simulink model "L4_SIM"  (R2018a)
settings: Solver=ode1  StartTime=0.0  StopTime=60  FixedStep=GLB_FIXED_STEP_SIZE_CPV  RelTol=1e-3  EnableMultiTasking=on
undefined symbols (not defined in the file or in its folder): Cf, Chassis, Cr, CYCLE_ACC1_2A__AdaptiveCruiseCtrlMode, CYCLE_ACC1_2A__AdaptiveCruiseCtrlSetSpeed, CYCLE_CCVS1_00__CruiseCtrlSetSpeed, CYCLE_CCVS1_00__WheelBasedVehicleSpeed, CYCLE_EEC1_00__EngSpeed, CYCLE_ETC1_00__TransDrivelineEngaged, CYCLE_ETC2_00__TransActualGearRatio, CYCLE_ETC7_03__TransMode1Indicator, CYCLE_GPS_Latitude, CYCLE_GPS_Longitude, CYCLE_LFE1_00__EngFuelRate, CYCLE_Net_Engine_Percent_Torque, CYCLE_SSI2_03__PitchAngleExRange, CYCLE_TIME, CYCLE_UTM_Origin_X, CYCLE_UTM_Origin_Y, CYCLE_Vehicle_Distance, DiscIntNeverNeededParam, ENUM_J1939_PCC_STATE_T, ENUM_J1939_SWITCH_T, ENUM_STEERING_WHEEL_ANGLE_SENSOR_TYPE_T, GLB_FIXED_STEP_SIZE_CPV, GLB_TRANS_LOSS_TRQ_GEAR_STEP_MPV, GLB_TRANS_LOSS_TRQ_SPD_STEP_MPV, GLB_TRANS_LOSS_TRQ_TABLE_DATA_MPV, GLB_TRANS_LOSS_TRQ_TRQ_STEP_MPV, GLB_VEHICLE_CONFIG_ACCEL_PED_GATEWAY_APV, heading_0, Iz, L4_Controller, lf, lr, position_0, ptc_matlab_lib, STEERCTRL_10ms, SUB_ECU_L4_MABX, SUB_L4_Task_10ms, SUB_L4_Task_10ms_SUB_STEERCTRL, SUB_PLANT_Chassis, Task_10ms, Vx_0
libraries: EmE_MBD_Blockset x81, PTC_MBDS_LIB x71, simulink x38, simulink_extras x1, SUB_L4_Task_10000ms x1, SUB_L4_Task_1000ms x1, SUB_L4_Task_100ms x1, SUB_L4_Task_10ms_SUB_APTC x1, SUB_L4_Task_10ms_SUB_BRKPEDARB x1, SUB_L4_Task_10ms_SUB_FAULT_MANAGER x1, SUB_L4_Task_10ms_SUB_STATE_CONTROL x1, simulink_need_slupdate x1
(part 2 of 6)

== system L4_SIM/Controllers/Virtual_Controllers/VECU ==
  In1 : Inport
  Bus Creator1 : BusCreator  Inputs=1
  Bus Creator2 : BusCreator  Inputs=2
  Constant1 : Constant  Value=0
  Constant2 : Constant  Value=0
  Terminator : Terminator
  Out1 : Outport
  wires:
  Bus Creator1/1 -> Out1/1
  In1/1 -> Terminator/1
  Bus Creator2/1 -> Bus Creator1/1  "TSC1_P4_VECU"
  Constant2/1 -> Bus Creator2/2  "TrqReq"
  Constant1/1 -> Bus Creator2/1  "OCM"

== system L4_SIM/Controllers/Virtual_Controllers/VEMC ==
  In1 : Inport
  Bus Creator1 : BusCreator  Inputs=3
  Bus Creator2 : BusCreator  Inputs=2
  Bus Creator3 : BusCreator  Inputs=2
  Constant{1..4} (4 alike) : Constant  Value=0
  Constant5 : Constant  Value=false
  Terminator : Terminator
  Out1 : Outport
  wires:
  Bus Creator1/1 -> Out1/1
  In1/1 -> Terminator/1
  Bus Creator2/1 -> Bus Creator1/1  "TSC1_P2_VEMCE"
  Constant2/1 -> Bus Creator2/2  "TrqReqE"
  Constant1/1 -> Bus Creator2/1  "OCME"
  Constant3/1 -> Bus Creator3/1  "OCMR"
  Constant4/1 -> Bus Creator3/2  "TrqReqR"
  Bus Creator3/1 -> Bus Creator1/2  "TSC1_P32_VEMCR"
  Constant5/1 -> Bus Creator1/3  "NeutralCoastRequest"

== system L4_SIM/Plant/PlantModel/Chassis ==
  Engine : Inport
  FoundationBrakes : Inport  Port=2
  AMT : Inport  Port=3
  Cycle : Inport  Port=4
  ABS : Inport  Port=5
  L4_MABX : Inport  Port=6
  Navigation : Inport  Port=7
  Bus Creator : BusCreator  Inputs=51
  Bus Selector : BusSelector  OutputSignals=EngineFricTrq,EngineIndicatedTrq,RetarderActTrqDem,RetarderTrqMax,EngFuelRate_lph,EngineIndicatedTrqMax,EngActNetTrqPer,EngActFricTrqPer,EngActIndTrqPer
  Bus Selector1 : BusSelector  OutputSignals=PitchAngle
  Bus Selector2 : BusSelector  OutputSignals=ShiftControl.Internal.GearNumberCommand,ShiftControl.Internal.MainClutch
  Bus Selector3 : BusSelector  OutputSignals=AeroDragForce,InclineForce,TireDragForce,TireResistancePower,RetarderNetTrq,RetarderPercentTrq,VehAccel,Vy,Yaw Rate
  Bus Selector4 : BusSelector  OutputSignals=ABS_VEHICLE_MASS_APV
  Bus Selector5 : BusSelector  OutputSignals=10msTask.SteeringControl.DesSteeringAngle
  Bus Selector6 : BusSelector  OutputSignals=Navigation.VehHeading
  Chassis_SL : Subsystem
  Constant : PTC_MBDS_LIB/Extras/Sources/Constant  Value2=GLB_AIR_DENSITY_APV  PTC_MBDS_BlockVersion=5.41  PTC_BlockType=PTC_MBDS_Constant
      settings: SourceProductName=PACCAR Technical Center MBDS Library
      settings: AttributesFormatString=|
      | Value: 1.23696005344
      | Unit: 'kg/m^3'
  Constant1 : PTC_MBDS_LIB/Extras/Sources/Constant  Value2=GLB_AXLE_EFFICIENCY_APV  PTC_MBDS_BlockVersion=5.41  PTC_BlockType=PTC_MBDS_Constant
      settings: SourceProductName=PACCAR Technical Center MBDS Library
      settings: AttributesFormatString=|
      | Value: 0.980000019073
      | Unit: '1'
  Constant11 : Constant  Value=[1,0]
  Constant2 : Constant  Value=[0 0]
  Constant3 : PTC_MBDS_LIB/Extras/Sources/Constant  Value2=GLB_CHASSIS_DRAG_COEFFICIENT_APV  PTC_MBDS_BlockVersion=5.41  PTC_BlockType=PTC_MBDS_Constant
      settings: SourceProductName=PACCAR Technical Center MBDS Library
      settings: AttributesFormatString=|
      | Value: 0.65
      | Unit: '1'
  Constant4 : Constant  Value=0
  Constant5 : Constant
  Constant9 : Constant  Value=[1,0]
  SignalConversion1 : SignalConversion  ConversionOutput=Contiguous copy  OverrideOpt=off
  SignalConversion3 : SignalConversion  ConversionOutput=Contiguous copy  OverrideOpt=off
  ChassisMdl_O : Outport
  wires:
  Bus Selector5/1 -> Chassis_SL/15(SteerAngle)  "<DesSteeringAngle>"
  L4_MABX/1 -> Bus Selector5/1
  Bus Selector3/9 -> Bus Creator/30  "<Yaw Rate>"
  Bus Selector3/8 -> Bus Creator/29  "<Vy>"
  Chassis_SL/28(BrakeSecondaryPressure_kpa) -> Bus Creator/36  "BrakeSecondaryPressure_kpa"
  Chassis_SL/27(BrakePrimaryPressure_kpa) -> Bus Creator/35  "BrakePrimaryPressure_kpa"
  Chassis_SL/26(BrakeApplicationPressure_kpa) -> Bus Creator/34  "BrakeApplicationPressure_kpa"
  Constant4/1 -> Chassis_SL/8(MotorTorqueRequest)
  SignalConversion1/1 -> Bus Creator/44  "EngineTorque_in"
  SignalConversion3/1 -> Bus Creator/43  "EngineFriction_In"
  Bus Selector/9 -> Bus Creator/51  "<EngActIndTrqPer>"
  Chassis_SL/21(VEHICLE_SPEED_OUT) -> Bus Creator/21  "VehicleSpeed"
  Chassis_SL/15(TRANSMISSION_SPEED_OUT) -> Bus Creator/15  "TransmissionSpeed"
  Bus Selector4/1 -> Chassis_SL/14(VehicleMass)  "<ABS_VEHICLE_MASS_APV>"
  ABS/1 -> Bus Selector4/1
  Constant/1 -> Chassis_SL/1(AirDensity)  "GLB_AIR_DENSITY_APV"
  Bus Selector/6 -> Bus Creator/48  "<EngineIndicatedTrqMax>"
  Bus Selector3/3 -> Bus Creator/24  "<TireDragForce>"
  Bus Selector/5 -> Bus Creator/47  "<EngFuelRate_lph>"
  Bus Selector3/7 -> Bus Creator/28  "<VehAccel>"
  Bus Selector/4 -> Bus Creator/46  "<RetarderTrqMax>"
  Bus Selector/3 -> Bus Creator/45  "<RetarderActTrqDem>"
  Bus Selector3/6 -> Bus Creator/27  "<RetarderPercentTrq>"
  Bus Selector/2 -> SignalConversion1/1  "<EngineIndicatedTrq>"
  Bus Selector/1 -> SignalConversion3/1  "<EngineFricTrq>"
  [Engine] -> Bus Selector/1
  Engine/1 -> Chassis_SL/7(EngineData), [Engine]
  Bus Selector3/5 -> Bus Creator/26  "<RetarderNetTrq>"
  Bus Selector3/4 -> Bus Creator/25  "<TireResistancePower>"
  Bus Selector3/2 -> Bus Creator/23  "<InclineForce>"
  Bus Selector3/1 -> Bus Creator/22  "<AeroDragForce>"
  Chassis_SL/22(DataBus) -> Bus Selector3/1  "ChassisDynamics"
  Chassis_SL/2(AXLE_SPEEDS_OUT[4]) -> Bus Creator/2  "AxleSpeeds"
  Bus Selector/8 -> Bus Creator/50  "<EngActFricTrqPer>"
  Bus Selector/7 -> Bus Creator/49  "<EngActNetTrqPer>"
  [FoundationBrakes] -> Bus Creator/37  "FoundationBrakes"
  FoundationBrakes/1 -> Chassis_SL/4(Brakes_Act), [FoundationBrakes]  "BrkDrv"
  AMT/1 -> Bus Selector2/1
  Bus Selector1/1 -> Chassis_SL/11(RoadAngle), Bus Creator/40  "<PitchAngle>"
  Cycle/1 -> Bus Selector1/1
  Chassis_SL/17(TRANSMISSION_TORQUE_OUT) -> Bus Creator/17  "TransmissionTorque"
  Chassis_SL/16(TRANSMISSION_STATE_LOCK_OUT) -> Bus Creator/16  "TransmissionStateLock"
  Chassis_SL/13(MEASURED_VEHICLE_SPEED_OUT) -> Bus Creator/13  "MeasuredVehicleSpeed_kph"
  Chassis_SL/12(MAIN_CLUTCH_LOCK_OUT) -> Bus Creator/12  "MainClutchLock"
  Chassis_SL/10(GEAR_NUMBER_OUT) -> Bus Creator/10  "GearNumber"
  Chassis_SL/9(ENGINE_RPM_OUT) -> Bus Creator/9  "EngineRPM"
  Chassis_SL/1(AXLE_POWER_LOSSES_OUT[2]) -> Bus Creator/1  "AxlePowerLosses"
  Bus Creator/1 -> ChassisMdl_O/1
  Bus Selector2/2 -> Chassis_SL/10(MainClutchAct), Bus Creator/39  "<MainClutch>"
  Constant2/1 -> Bus Creator/41, Chassis_SL/12(TransmissionLoss[2])  "TransmisisonLoss_In"
  Constant11/1 -> Bus Creator/42, Chassis_SL/13(TransmissionSpinLoss[2])  "TransSpinLoss_In"
  Constant9/1 -> Chassis_SL/6(DriveShaftLoss[2])
  Constant3/1 -> Chassis_SL/5(C_Drag)  "GLB_CHASSIS_DRAG_COEFFICIENT_APV"
  Constant5/1 -> Chassis_SL/3(Axle_Act_Lock)
  Constant1/1 -> Chassis_SL/2(AxleEff)  "GLB_AXLE_EFFICIENCY_APV"
  Chassis_SL/14(TRANSMISSION_POWER_LOSS_OUT) -> Bus Creator/14  "TransmissionPowerLoss"
  Chassis_SL/8(DRIVE_SHAFT_TORQUE_OUT) -> Bus Creator/8  "DriveShaftTorque"
  Chassis_SL/20(BrakeTrqRequest) -> Bus Creator/20  "ChassisBrakeTrqRequest"
  Chassis_SL/6(DRIVE_SHAFT_POWER_LOSS_OUT) -> Bus Creator/6  "DrIveShaftPowerLoss"
  Chassis_SL/18(TRANS_SPIN_POWER_LOSS_OUT) -> Bus Creator/18  "TransmissionSpinPowerLoss"
  Chassis_SL/4(BRAKES_LOCK_OUT[4]) -> Bus Creator/4  "BrakesLock"
  Chassis_SL/7(DRIVE_SHAFT_SPEED_OUT) -> Bus Creator/7  "DriveShaftSpeed"
  Chassis_SL/19(TRANS_SPIN_SPEED_OUT) -> Bus Creator/19  "TransmissionSpinSpeed"
  Chassis_SL/3(AXLE_TORQUES_OUT[2]) -> Bus Creator/3  "AxleTorques"
  Chassis_SL/11(GEAR_RATIO_OUT) -> Bus Creator/11  "GearRatio"
  Chassis_SL/5(DRIVE_AXLE_LOCK_OUT) -> Bus Creator/5  "DriveAxleLock"
  Bus Selector2/1 -> Bus Creator/38, Chassis_SL/9(GearNumber)  "<GearNumberCommand>"
  Chassis_SL/23(TrqFromClutch) -> Bus Creator/31  "TrqFromClutch"
  Chassis_SL/24(ClutchState) -> Bus Creator/32  "ClutchState"
  Chassis_SL/25(EngSpdClutchClosed) -> Bus Creator/33  "EngSpdClutchClosed"
  Navigation/1 -> Bus Selector6/1
  Bus Selector6/1 -> Chassis_SL/16(Heading)  "<VehHeading>"

== system L4_SIM/Plant/PlantModel/Navigation ==
  In1 : Inport
  Body velocity : Scope  NumInputPorts=2
  Bus Creator : BusCreator  Inputs=3
  Bus Selector : BusSelector  OutputSignals=VehicleSpeed,Vy,Yaw Rate
  Gain : Gain  Gain=180/pi
  Gain1 : Gain  Gain=1/3.6
  Heading : Scope  NumInputPorts=2
  Initial Heading : Constant  Value=heading_0
  Initial Position : Constant  Value=position_0
  Integrator : Integrator  InitialConditionSource=external
  Integrator2 : Integrator  InitialCondition=heading_0  UpperSaturationLimit=pi  LowerSaturationLimit=-pi  WrapState=on  WrappedStateUpperValue=2*pi  WrappedStateLowerValue=0
  MATLAB Function1 : MATLAB Function  TreatAsAtomicUnit=on
  Position : Scope
  Yaw rate : Scope
  Out1 : Outport
  wires:
  Gain1/1 -> MATLAB Function1/1(Vx), Body velocity/1
  Integrator2/1 -> MATLAB Function1/3(heading), Gain/1, Heading/1
  Gain/1 -> Bus Creator/3  "VehHeading"
  Integrator/1 -> Bus Creator/2, Position/1  "VehPosition"
  Bus Creator/1 -> Out1/1
  Initial Heading/1 -> Heading/2
  Initial Position/1 -> Integrator/2
  MATLAB Function1/1(Vnav) -> Integrator/1, Bus Creator/1  "VehVelNav"
  Bus Selector/2 -> MATLAB Function1/2(Vy), Body velocity/2  "<Vy>"
  Bus Selector/1 -> Gain1/1  "<VehicleSpeed>"
  Bus Selector/3 -> Integrator2/1, Yaw rate/1  "<Yaw Rate>"
  In1/1 -> Bus Selector/1

== system L4_SIM/Controllers/Drive_Cycle/DriveCycle/CruiseSetSpeedOverride ==
  SimActiveTime : Inport
  CCSetSpeed : Inport  Port=2
  Constant1 : PTC_MBDS_LIB/Extras/Sources/Constant  Value2=60  PTC_MBDS_BlockVersion=5.41  PTC_BlockType=PTC_MBDS_Constant
      settings: SourceProductName=PACCAR Technical Center MBDS Library
  Constant2 : PTC_MBDS_LIB/Extras/Sources/Constant  Value2=0  PTC_MBDS_BlockVersion=5.41  PTC_BlockType=PTC_MBDS_Constant
      settings: SourceProductName=PACCAR Technical Center MBDS Library
  Display : Display
  Display1 : Display
  If_Then_Else1 : PTC_MBDS_LIB/Extras/Signal Routing/If_Then_Else  PTC_MBDS_BlockVersion=5.41  PTC_BlockType=PTC_MBDS_If_Then_Else
      settings: SourceProductName=PACCAR Technical Center MBDS Library
  LE : PTC_MBDS_LIB/MBDS Standard Library/Basic Operations/Logic and Bit Operations/LE  InputSameDT=on  PTC_MBDS_BlockVersion=5.41  PTC_BlockType=PTC_MBDS_LE
      settings: SourceProductName=PACCAR Technical Center MBDS Library
  Out1 : Outport
  wires:
  Constant1/1 -> LE/2
  CCSetSpeed/1 -> If_Then_Else1/3
  SimActiveTime/1 -> Display/1, LE/1
  Constant2/1 -> If_Then_Else1/2
  If_Then_Else1/1 -> Display1/1, Out1/1
  LE/1 -> If_Then_Else1/1

== system L4_SIM/Controllers/Drive_Cycle/DriveCycle/CycleCalculations ==
  Actual_Vehicle_Speed[m/s] : Inport
  Discrete-Time Integrator : DiscreteIntegrator  IntegratorMethod=Integration: Trapezoidal  SampleTime=-1  ICPrevOutput=DiscIntNeverNeededParam  ICPrevScaledInput=DiscIntNeverNeededParam
  Saturation : Saturate  UpperLimit=Inf  LowerLimit=0
  Vehicle_Distance[m] : Outport
  wires:
  Actual_Vehicle_Speed[m/s]/1 -> Saturation/1
  Discrete-Time Integrator/1 -> Vehicle_Distance[m]/1
  Saturation/1 -> Discrete-Time Integrator/1

== system L4_SIM/Controllers/Operator/Subsystem/Gains ==
  note: These Gains should be the same for Acc Pedal
      | and Brake Pedal on the dyno
  Constant : PTC_MBDS_LIB/Extras/Sources/Constant  Value2=OPERATOR_Kp_Acc  PTC_MBDS_BlockVersion=5.41  PTC_BlockType=PTC_MBDS_Constant
      settings: SourceProductName=PACCAR Technical Center MBDS Library
      settings: AttributesFormatString=|
      | Value: 0.25
      | Unit: '1'
  Constant1 : PTC_MBDS_LIB/Extras/Sources/Constant  Value2=OPERATOR_Ti_Acc  PTC_MBDS_BlockVersion=5.41  PTC_BlockType=PTC_MBDS_Constant
      settings: SourceProductName=PACCAR Technical Center MBDS Library
      settings: AttributesFormatString=|
      | Value: 0.45
      | Unit: 's'
  Constant2 : PTC_MBDS_LIB/Extras/Sources/Constant  Value2=OPERATOR_Td_Acc  PTC_MBDS_BlockVersion=5.41  PTC_BlockType=PTC_MBDS_Constant
      settings: SourceProductName=PACCAR Technical Center MBDS Library
      settings: AttributesFormatString=|
      | Value: 0
      | Unit: 's'
  Constant3 : PTC_MBDS_LIB/Extras/Sources/Constant  Value2=OPERATOR_Kp_Brk  PTC_MBDS_BlockVersion=5.41  PTC_BlockType=PTC_MBDS_Constant
      settings: SourceProductName=PACCAR Technical Center MBDS Library
      settings: AttributesFormatString=|
      | Value: 0.38
      | Unit: '1'
  Constant4 : PTC_MBDS_LIB/Extras/Sources/Constant  Value2=OPERATOR_Ti_Brk  PTC_MBDS_BlockVersion=5.41  PTC_BlockType=PTC_MBDS_Constant
      settings: SourceProductName=PACCAR Technical Center MBDS Library
      settings: AttributesFormatString=|
      | Value: 0.25
      | Unit: 's'
  Constant5 : PTC_MBDS_LIB/Extras/Sources/Constant  Value2=OPERATOR_Td_Brk  PTC_MBDS_BlockVersion=5.41  PTC_BlockType=PTC_MBDS_Constant
      settings: SourceProductName=PACCAR Technical Center MBDS Library
      settings: AttributesFormatString=|
      | Value: 0
      | Unit: 's'
  Mux : Mux  Inputs=3
  Mux1 : Mux  Inputs=3
  Gains_Acc : Outport
  Gains_Brk : Outport  Port=2
  wires:
  Mux1/1 -> Gains_Brk/1
  Constant3/1 -> Mux1/1  "OPERATOR_Kp_Brk"
  Constant4/1 -> Mux1/2  "OPERATOR_Ti_Brk"
  Constant5/1 -> Mux1/3  "OPERATOR_Td_Brk"
  Mux/1 -> Gains_Acc/1
  Constant2/1 -> Mux/3  "OPERATOR_Td_Acc"
  Constant1/1 -> Mux/2  "OPERATOR_Ti_Acc"
  Constant/1 -> Mux/1  "OPERATOR_Kp_Acc"

== system L4_SIM/Controllers/Operator/Subsystem/HeadingController ==
  <VehPosition> : Inport
  <Waypoint> : Inport  Port=2
  Demux : Demux  Outputs=2
  Heading : Scope
  MATLAB Function : MATLAB Function  TreatAsAtomicUnit=on
  Position : Scope  NumInputPorts=2
  XY Graph : simulink/Sinks/XY Graph  xmin=-100  xmax=100  ymin=-100  ymax=100  st=-1
  rad2deg : Gain  Gain=180/pi
  TargetHeading : Outport
  wires:
  Demux/2 -> MATLAB Function/2(yN), XY Graph/2
  rad2deg/1 -> TargetHeading/1
  <VehPosition>/1 -> Position/2, Demux/1
  <Waypoint>/1 -> Position/1, MATLAB Function/3(target_waypoint)
  MATLAB Function/1(heading) -> Heading/1, rad2deg/1
  Demux/1 -> MATLAB Function/1(xN), XY Graph/1

== system L4_SIM/Controllers/Operator/Subsystem/PedalArbitration ==
  PedGov : Inport
  BrkGov : Inport  Port=2
  VehSpdAct : Inport  Port=3
  VehSpdTarget : Inport  Port=4
  CCSetSpd : Inport  Port=5
  Constant : Constant
  Constant1 : Constant  Value=0
  Constant2 : Constant  Value=-1
  Constant3 : Constant  Value=0
  Constant4 : Constant  Value=20
  Detect Increase : simulink/Logic and Bit Operations/Detect Increase  RequirementInfo={} %GIDa_5b363545_e358_46c0_be1c_cb20273c47ec  vinit=0.0  OutDataTypeStr=boolean
  Detect Increase1 : simulink/Logic and Bit Operations/Detect Increase  RequirementInfo={} %GIDa_08716cdf_9875_4430_a2e6_6acea910ba87  vinit=0.0  OutDataTypeStr=boolean
  Logical Operator : Logic  Operator=NOT  AllPortsSameDT=off  OutDataTypeStr=boolean
  Logical Operator1 : Logic  Operator=OR  AllPortsSameDT=off  OutDataTypeStr=boolean
  Logical Operator2 : Logic  Operator=OR  AllPortsSameDT=off  OutDataTypeStr=boolean
  Logical Operator3 : Logic  Operator=NOT  AllPortsSameDT=off  OutDataTypeStr=boolean
  Logical Operator4 : Logic  AllPortsSameDT=off  OutDataTypeStr=boolean
  Logical Operator5 : Logic  AllPortsSameDT=off  OutDataTypeStr=boolean
  Relational Operator : RelationalOperator  OutDataTypeStr=boolean  RndMeth=Nearest
  Relational Operator1 : RelationalOperator  OutDataTypeStr=boolean  RndMeth=Nearest
  Relational Operator2 : RelationalOperator  Operator=<=  OutDataTypeStr=boolean  RndMeth=Nearest
  Relational Operator3 : RelationalOperator  OutDataTypeStr=boolean  RndMeth=Nearest
  S-R Flip-Flop : simulink_extras/Flip Flops/S-R Flip-Flop  RequirementInfo={} %GIDa_30642f6b_cc04_4a68_bd17_75a151f00dc4  initial_condition=0
  Subtract : Sum  Inputs=+-
  Switch : Switch  Criteria=u2 ~= 0
  Switch1 : Switch  Criteria=u2 ~= 0
  Terminator : Terminator
  BrkDrv : Outport
  PedDrv : Outport  Port=2
  EngSpdGovReset : Outport  Port=3
  BrakeSpdGovReset : Outport  Port=4
  wires:
  Relational Operator2/1 -> Logical Operator2/1
  Logical Operator2/1 -> S-R Flip-Flop/2
  Constant4/1 -> Relational Operator3/2, Relational Operator/2
  Detect Increase1/1 -> BrakeSpdGovReset/1
  Detect Increase/1 -> EngSpdGovReset/1
  Constant2/1 -> Relational Operator2/2
  Logical Operator1/1 -> Logical Operator/1
  Relational Operator1/1 -> S-R Flip-Flop/1
  Constant/1 -> Relational Operator1/2
  Subtract/1 -> Relational Operator1/1, Relational Operator2/1
  VehSpdTarget/1 -> Subtract/2
  VehSpdAct/1 -> Relational Operator/1, Subtract/1
  PedGov/1 -> Switch/1
  Switch1/1 -> BrkDrv/1
  Switch/1 -> PedDrv/1
  Logical Operator/1 -> Switch/2, Detect Increase/1
  BrkGov/1 -> Switch1/1
  Constant3/1 -> Switch1/3
  S-R Flip-Flop/1 -> Logical Operator1/1, Logical Operator4/1, Detect Increase1/1
  Constant1/1 -> Switch/3
  Logical Operator3/1 -> Logical Operator4/2
  Logical Operator4/1 -> Switch1/2
  S-R Flip-Flop/2 -> Terminator/1
  CCSetSpd/1 -> Relational Operator3/1
  Relational Operator/1 -> Logical Operator5/1
  Relational Operator3/1 -> Logical Operator5/2
  Logical Operator5/1 -> Logical Operator1/2, Logical Operator3/1, Logical Operator2/2

== system L4_SIM/Controllers/Operator/Subsystem/SpdControlBrake ==
  VehSpdTarget : Inport
  VehSpdAct : Inport  Port=2
  Gains : Inport  Port=3
  Reset : Inport  Port=4
  Demux : Demux  Outputs=3
  SpdControlBrake : Subsystem
  BrakeComGov(0-1) : Outport
  wires:
  Reset/1 -> SpdControlBrake/6(Reset)
  SpdControlBrake/1(BrakeComGov(0-1)) -> BrakeComGov(0-1)/1
  Gains/1 -> Demux/1
  Demux/3 -> SpdControlBrake/5(Td)
  Demux/2 -> SpdControlBrake/4(Ti)
  Demux/1 -> SpdControlBrake/3(Kp)
  VehSpdAct/1 -> SpdControlBrake/2(VehSpdAct)
  VehSpdTarget/1 -> SpdControlBrake/1(VehSpdTarget)

== system L4_SIM/Controllers/Operator/Subsystem/SpdControlTraction ==
  VehSpdTarget : Inport
  VehSpdAct : Inport  Port=2
  Gains : Inport  Port=3
  Reset : Inport  Port=4
  Demux : Demux  Outputs=3
  SpdControlTraction : Subsystem
  PedalComGov(0-1) : Outport
  wires:
  Reset/1 -> SpdControlTraction/6(Reset)
  SpdControlTraction/1(PedalComGov(0-1)) -> PedalComGov(0-1)/1
  Gains/1 -> Demux/1
  Demux/3 -> SpdControlTraction/5(Td)
  Demux/2 -> SpdControlTraction/4(Ti)
  Demux/1 -> SpdControlTraction/3(Kp)
  VehSpdAct/1 -> SpdControlTraction/2(VehSpdAct)
  VehSpdTarget/1 -> SpdControlTraction/1(VehSpdTarget)

== system L4_SIM/Controllers/Virtual_Controllers/ABS/ConvertRPM2kph ==
  <AxleSpeeds> : Inport  Unit=rpm
  Constant7 : PTC_MBDS_LIB/Extras/Sources/Constant  Value2=GLB_TIRE_DIAMETER_APV  PTC_MBDS_BlockVersion=5.41  PTC_BlockType=PTC_MBDS_Constant
      settings: SourceProductName=PACCAR Technical Center MBDS Library
      settings: AttributesFormatString=|
      | Value: 1
      | Unit: 'm'
  Product : Product
  km/meter : Gain  Gain=1/1000
  minutes/hour : Gain  Gain=60
  pi : Gain  Gain=pi
  Spd : Outport  Unit=km/h
  wires:
  pi/1 -> Product/2
  Constant7/1 -> pi/1  "GLB_TIRE_DIAMETER_APV"
  <AxleSpeeds>/1 -> Product/1
  Product/1 -> minutes/hour/1
  minutes/hour/1 -> km/meter/1
  km/meter/1 -> Spd/1

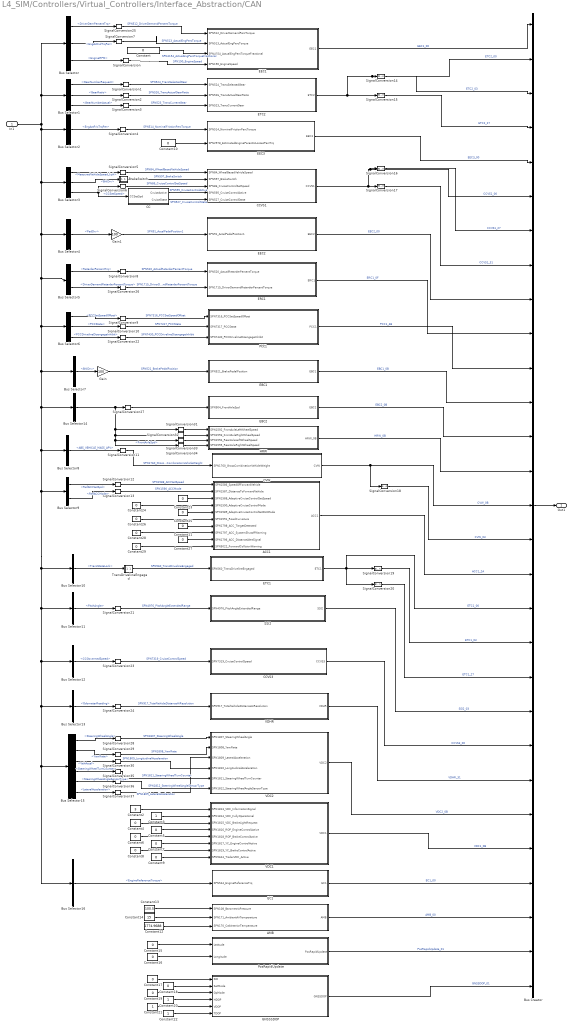
== system L4_SIM/Controllers/Virtual_Controllers/Interface_Abstraction/CAN ==
  In1 : Inport
  ACC1 : Subsystem
  AMB : Subsystem
  BrakeSwitch : Subsystem
  Bus Creator : BusCreator  Inputs=29
  Bus Selector : BusSelector  OutputSignals=Feedback_controllers.PCI.DriverDemPercentTrq,Feedback_sensors.Chassis.EngActIndTrqPer,Feedback_sensors.Chassis.EngineRPM
  Bus Selector1 : BusSelector  OutputSignals=Feedback_controllers.AMT.ShiftControl.External.GearNumberRequest,Feedback_sensors.Chassis.GearRatio,Feedback_controllers.AMT.ShiftControl.External.GearNumberActual
  Bus Selector10 : BusSelector  OutputSignals=Feedback_controllers.AMT.ShiftControl.External.TransStateLock
  Bus Selector11 : BusSelector  OutputSignals=Cycle.PitchAngle
  Bus Selector12 : BusSelector  OutputSignals=Feedback_controllers.PCI.CCData.CCGovernedSpeed
  Bus Selector13 : BusSelector  OutputSignals=Cycle.OdometerReading
  Bus Selector14 : BusSelector  OutputSignals=Feedback_controllers.ABS.FrontAxleSpd
  Bus Selector15 : BusSelector  OutputSignals=Feedback_controllers.ABS.SteeringWheelAngle,Feedback_controllers.ABS.YawRate,Feedback_sensors.Chassis.VehAccel,Feedback_controllers.ABS.SteeringWheelTurnCounter,Feedback_controllers.ABS.SteeringWheelAngleSensorType,Feedback_controllers.ABS.LateralAcceleration
  Bus Selector16 : BusSelector  OutputSignals=Feedback_controllers.PCI.CCData.EngineReferenceTorque
  Bus Selector2 : BusSelector  OutputSignals=Feedback_sensors.Engine.EngActFricTrqPer
  Bus Selector3 : BusSelector  OutputSignals=Feedback_sensors.Chassis.MeasuredVehicleSpeed_kph,Operator.BrkDrv,Cycle.CCSetSpeed
  Bus Selector4 : BusSelector  OutputSignals=Operator.PedDrv
  Bus Selector5 : BusSelector  OutputSignals=Feedback_sensors.Chassis.RetarderPercentTrq,Feedback_controllers.PCI.CCData.DriverDemandRetarderPercentTorque
  Bus Selector6 : BusSelector  OutputSignals=Feedback_controllers.PCC.PCCSetSpeedOffset,Feedback_controllers.PCC.PCCState,Feedback_controllers.PCC.PCCDrivelineDisengageInhibit
  Bus Selector7 : BusSelector  OutputSignals=Operator.BrkDrv
  Bus Selector8 : BusSelector  OutputSignals=Feedback_controllers.ABS.ABS_VEHICLE_MASS_APV
  Bus Selector9 : BusSelector  OutputSignals=Cycle.RefACCSetSpd,Cycle.RefACCMode
  CC : Subsystem
  CCVS1 : Subsystem
  CCVS3 : Subsystem
  CVW : Subsystem
  Constant{,4..11,15..19,23..29} (21 alike) : Constant  Value=0
  Constant12 : Constant  Value=1774.9688
  Constant13 : Constant  Value=100.5
  Constant14 : Constant  Value=15
  Constant2 : Constant  Value=3
  Constant{3,20..22} (4 alike) : Constant
  EBC1 : Subsystem
  EBC2 : Subsystem
  EC1 : Subsystem
  EEC1 : Subsystem
  EEC2 : Subsystem
  EEC3 : Subsystem
  ERC1 : Subsystem
  ETC1 : Subsystem
  ETC2 : Subsystem
  GNSSSDOP : Subsystem
  Gain : Gain  Gain=100
  Gain1 : Gain  Gain=100
  HRW : Subsystem
  PCC1 : Subsystem
  PosRapidUpdate : Subsystem
  SSI2 : Subsystem
  SignalConversion{,1..37} (38 alike) : SignalConversion  ConversionOutput=Contiguous copy  OverrideOpt=off
  TransDrivelineEngaged : Subsystem
  VDC1 : Subsystem
  VDC2 : Subsystem
  VDHR : Subsystem
  Out1 : Outport
  wires:
  Bus Selector3/3 -> SignalConversion6/1, CC/1(CCSetSpd)  "<CCSetSpeed>"
  In1/1 -> Bus Selector14/1, Bus Selector16/1, Bus Selector15/1, Bus Selector13/1, Bus Selector12/1, Bus Selector11/1, Bus Selector10/1, Bus Selector9/1, Bus Selector8/1, Bus Selector7/1, Bus Selector6/1, Bus Selector5/1, Bus Selector4/1, Bus Selector3/1, Bus Selector2/1, Bus Selector/1, Bus Selector1/1
  Bus Selector/3 -> SignalConversion/1  "<EngineRPM>"
  Bus Selector5/1 -> SignalConversion8/1  "<RetarderPercentTrq>"
  Bus Selector/2 -> SignalConversion7/1  "<EngActIndTrqPer>"
  Bus Selector1/3 -> SignalConversion3/1  "<GearNumberActual>"
  SignalConversion5/1 -> CCVS1/1(SPN84_WheelBasedVehicleSpeed)  "SPN84_WheelBasedVehicleSpeed"
  Bus Selector2/1 -> SignalConversion4/1  "<EngActFricTrqPer>"
  SignalConversion4/1 -> EEC3/1(SPN514_NominalFrictionPercTorque)  "SPN514_NominalFrictionPercTorque"
  Constant/1 -> EEC1/3(SPN4154_ActualEngPercTorqueFractional)  "SPN4154_ActualEngPercTorqueFractional"
  SignalConversion2/1 -> ETC2/2(SPN526_TransActualGearRatio)  "SPN526_TransActualGearRatio"
  SignalConversion/1 -> EEC1/4(SPN190_EngineSpeed)  "SPN190_EngineSpeed"
  Bus Selector3/1 -> SignalConversion5/1  "<MeasuredVehicleSpeed_kph>"
  BrakeSwitch/1(Out) -> CCVS1/2(SPN597_BrakeSwitch)  "SPN597_BrakeSwitch"
  SignalConversion1/1 -> ETC2/1(SPN524_TransSelectedGear)  "SPN524_TransSelectedGear"
  CC/1(CruiseActive) -> CCVS1/4(SPN595_CruiseControlActive)  "SPN595_CruiseControlActive"
  CC/2(CruiseState) -> CCVS1/5(SPN527_CruiseControlState)  "SPN527_CruiseControlState"
  Bus Selector4/1 -> Gain1/1  "<PedDrv>"
  Bus Selector3/2 -> BrakeSwitch/1(In)  "<BrkDrv>"
  Bus Selector1/2 -> SignalConversion2/1  "<GearRatio>"
  Bus Selector1/1 -> SignalConversion1/1  "<GearNumberRequest>"
  SignalConversion6/1 -> CCVS1/3(SPN86_CruiseControlSetSpeed)  "SPN86_CruiseControlSetSpeed"
  SignalConversion8/1 -> ERC1/1(SPN520_ActualRetarderPercentTorque)  "SPN520_ActualRetarderPercentTorque"
  SignalConversion7/1 -> EEC1/2(SPN513_ActualEngPercTorque)  "SPN513_ActualEngPercTorque"
  SignalConversion3/1 -> ETC2/3(SPN523_TransCurrentGear)  "SPN523_TransCurrentGear"
  Bus Creator/1 -> Out1/1
  Bus Selector6/1 -> SignalConversion9/1  "<PCCSetSpeedOffset>"
  Bus Selector6/2 -> SignalConversion10/1  "<PCCState>"
  Bus Selector7/1 -> Gain/1  "<BrkDrv>"
  Gain/1 -> EBC1/1(SPN521_BrakePedalPosition)  "SPN521_BrakePedalPosition"
  SignalConversion9/1 -> PCC1/1(SPN7316_PCCSetSpeedOffset)  "SPN7316_PCCSetSpeedOffset"
  SignalConversion10/1 -> PCC1/2(SPN7317_PCCState)  "SPN7317_PCCState"
  Bus Selector8/1 -> SignalConversion11/1  "<ABS_VEHICLE_MASS_APV>"
  SignalConversion12/1 -> ACC1/1(SPN1586_SpeedOfForwardVehicle)  "SPN1588_ACCSetSpeed"
  SignalConversion13/1 -> ACC1/2(SPN1587_DistanceToForwardVehicle)  "SPN1590_ACCMode"
  Bus Selector10/1 -> TransDrivelineEngaged/1(In1)  "<TransStateLock>"
  TransDrivelineEngaged/1(Out1) -> ETC1/1(SPN560_TransDrivelineEngaged)  "SPN560_TransDrivelineEngaged"
  EEC1/1(EEC1) -> Bus Creator/1  "EEC1_00"
  ETC2/1(ETC2) -> SignalConversion14/1, Bus Creator/2, SignalConversion15/1  "ETC2_00"
  SignalConversion14/1 -> Bus Creator/3  "ETC2_03"
  SignalConversion15/1 -> Bus Creator/4  "ETC2_27"
  EEC3/1(EEC3) -> Bus Creator/5  "EEC3_00"
  CCVS1/1(CCVS1) -> SignalConversion17/1, SignalConversion16/1, Bus Creator/6  "CCVS1_00"
  SignalConversion16/1 -> Bus Creator/7  "CCVS1_27"
  SignalConversion17/1 -> Bus Creator/8  "CCVS1_31"
  EEC2/1(EEC2) -> Bus Creator/9  "EEC2_00"
  ERC1/1(ERC1) -> Bus Creator/10  "ERC1_0F"
  PCC1/1(PCC1) -> Bus Creator/11  "PCC1_4B"
  EBC1/1(EBC1) -> Bus Creator/12  "EBC1_0B"
  CVW/1(CVW) -> Bus Creator/15, SignalConversion18/1  "CVW_0B"
  SignalConversion18/1 -> Bus Creator/16  "CVW_03"
  ACC1/1(ACC1) -> Bus Creator/17  "ACC1_2A"
  ETC1/1(ETC1) -> Bus Creator/18, SignalConversion20/1, SignalConversion19/1  "ETC1_00"
  SignalConversion19/1 -> Bus Creator/19  "ETC1_03"
  SignalConversion20/1 -> Bus Creator/20  "ETC1_27"
  Bus Selector11/1 -> SignalConversion21/1  "<PitchAngle>"
  SignalConversion21/1 -> SSI2/1(SPN4976_PitchAngleExtendedRange)  "SPN4976_PitchAngleExtendedRange"
  SSI2/1(SSI2) -> Bus Creator/21  "SSI2_03"
  Bus Selector6/3 -> SignalConversion22/1  "<PCCDrivelineDisengageInhibit>"
  SignalConversion22/1 -> PCC1/3(SPN7430_PCCDrivelineDisengageInhibit)  "SPN7430_PCCDrivelineDisengageInhibit"
  Bus Selector12/1 -> SignalConversion23/1  "<CCGovernedSpeed>"
  SignalConversion23/1 -> CCVS3/1(SPN7319_CruiseControlSpeed)  "SPN7319_CruiseControlSpeed"
  CCVS3/1(CCVS3) -> Bus Creator/22  "CCVS3_00"
  Bus Selector9/1 -> SignalConversion12/1  "<RefACCSetSpd>"
  Bus Selector9/2 -> SignalConversion13/1  "<RefACCMode>"
  Gain1/1 -> EEC2/1(SPN91_AccelPedalPosition1)  "SPN91_AccelPedalPosition1"
  Bus Selector13/1 -> SignalConversion24/1  "<OdometerReading>"
  SignalConversion24/1 -> VDHR/1(SPN917_TotalVehicleDistanceHiResolution)  "SPN917_TotalVehicleDistanceHiResolution"
  VDHR/1(VDHR) -> Bus Creator/23  "VDHR_31"
  Bus Selector/1 -> SignalConversion25/1  "<DriverDemPercentTrq>"
  SignalConversion25/1 -> EEC1/1(SPN512_DriverDemandPercTorque)  "SPN512_DriverDemandPercentTorque"
  Bus Selector5/2 -> SignalConversion26/1  "<DriverDemandRetarderPercentTorque>"
  SignalConversion26/1 -> ERC1/2(SPN1715_DriverDemandRetarderPercentTorque)  "SPN1715_DriverDemandRetarderPercentTorque"
  Bus Selector14/1 -> SignalConversion31/1, SignalConversion32/1, SignalConversion33/1, SignalConversion34/1, SignalConversion27/1  "<FrontAxleSpd>"
  SignalConversion27/1 -> EBC2/1(SPN904_FrontAxleSpd)
  EBC2/1(EBC2) -> Bus Creator/13  "EBC2_0B"
  VDC2/1(VDC2) -> Bus Creator/24  "VDC2_0B"
  Bus Selector15/1 -> SignalConversion28/1  "<SteeringWheelAngle>"
  Bus Selector15/2 -> SignalConversion29/1  "<YawRate>"
  SignalConversion28/1 -> VDC2/1(SPN1807_SteeringWheelAngle)  "SPN1807_SteeringWheelAngle"
  SignalConversion29/1 -> VDC2/2(SPN1808_YawRate)  "SPN1808_YawRate"
  Bus Selector15/3 -> SignalConversion30/1  "<VehAccel>"
  SignalConversion30/1 -> VDC2/4(SPN1810_LongitudinalAcceleration)  "SPN1809_LongitudinalAcceleration"
  Constant2/1 -> VDC1/1(SPN1813_VDC_InformationSignal)
  Constant3/1 -> VDC1/2(SPN1814_VDC_FullyOperational)
  Constant4/1 -> VDC1/3(SPN1815_VDC_BrakeLightRequest)
  Constant5/1 -> VDC1/4(SPN1816_ROP_EngineControlActive)
  Constant6/1 -> VDC1/5(SPN1818_ROP_BrakeControlActive)
  Constant7/1 -> VDC1/6(SPN1817_YC_EngineControlActive)
  Constant8/1 -> VDC1/7(SPN1819_YC_BrakeControlActive)
  Constant9/1 -> VDC1/8(SPN5624_TrailerVDC_Active)
  VDC1/1(VDC1) -> Bus Creator/25  "VDC1_0B"
  Constant10/1 -> EEC3/2(SPN2978_EstimatedEngineParasiticLossesPercTrq)
  Bus Selector16/1 -> EC1/1(SPN544_EngineReferenceTrq)  "<EngineReferenceTorque>"
  EC1/1(EC1) -> Bus Creator/26  "EC1_00"
  Constant12/1 -> AMB/3(SPN170_CabInteriorTemperature)
  Constant13/1 -> AMB/1(SPN108_BarometricPressure)
  Constant14/1 -> AMB/2(SPN171_AmbientAirTemperature)
  AMB/1(AMB) -> Bus Creator/27  "AMB_00"
  SignalConversion34/1 -> HRW/4(SPN1595_RearAxleRightWheelSpeed)
  SignalConversion33/1 -> HRW/3(SPN1594_RearAxleLeftWheelSpeed)
  SignalConversion32/1 -> HRW/2(SPN1593_FrontAxleRightWheelSpeed)
  SignalConversion31/1 -> HRW/1(SPN1592_FrontAxleLeftWheelSpeed)
  HRW/1(HRW_0B) -> Bus Creator/14  "HRW_0B"
  Constant15/1 -> PosRapidUpdate/1(Latitude)
  Constant16/1 -> PosRapidUpdate/2(Longitude)
  PosRapidUpdate/1(PosRapidUpdate) -> Bus Creator/28  "PosRapidUpdate_01"
  Constant22/1 -> GNSSSDOP/6(TDOP)
  Constant21/1 -> GNSSSDOP/5(VDOP)
  Constant20/1 -> GNSSSDOP/4(HDOP)
  Constant19/1 -> GNSSSDOP/3(OpMode)
  Constant18/1 -> GNSSSDOP/2(SetMode)
  Constant17/1 -> GNSSSDOP/1(SID)
  GNSSSDOP/1(GNSSDOP) -> Bus Creator/29  "GNSSDOP_01"
  Constant23/1 -> ACC1/3(SPN1588_AdaptiveCruiseControlSetSpeed)
  Constant24/1 -> ACC1/4(SPN1590_AdaptiveCruiseControlMode)
  Constant25/1 -> ACC1/5(SPN1589_AdaptiveCruiseControlSetDistMode)
  Constant26/1 -> ACC1/6(SPN1591_RoadCurvature)
  SignalConversion11/1 -> CVW/1(SPN1760_GrossCombinationVehicleWeight)  "SPN1760_GrossCombinationVehicleWeight"
  Constant11/1 -> ACC1/7(SPN1798_ACC_TargetDetected)
  Constant28/1 -> ACC1/8(SPN1797_ACC_SystemShutoffWarning)
  Constant27/1 -> ACC1/9(SPN1796_ACC_DistanceAlertSignal)
  Constant29/1 -> ACC1/10(SPN5022_ForwardCollisionWarning)
  Bus Selector15/4 -> SignalConversion35/1  "<SteeringWheelTurnCounter>"
  Bus Selector15/5 -> SignalConversion36/1  "<SteeringWheelAngleSensorType>"
  Bus Selector15/6 -> SignalConversion37/1  "<LateralAcceleration>"
  SignalConversion35/1 -> VDC2/5(SPN1811_SteeringWheelTurnCounter)  "SPN1811_SteeringWheelTurnCounter"
  SignalConversion36/1 -> VDC2/6(SPN1812_SteeringWheelAngleSensorType)  "SPN1812_SteeringWheelAngleSensorType"
  SignalConversion37/1 -> VDC2/3(SPN1809_LateralAcceleration)  "SPN1809_LateralAcceleration"

== system L4_SIM/Controllers/Virtual_Controllers/Interface_Abstraction/HW ==
  Inport : Inport
  Bus Creator : BusCreator  Inputs=2
  Bus Selector : BusSelector  OutputSignals=Feedback_controllers.L4_MABX.10msTask.APTC.APTC_arb_pedal_position,Operator.PedDrv
  Constant : Constant  Value=GLB_VEHICLE_CONFIG_ACCEL_PED_GATEWAY_APV
  If_Then_Else : EmE_MBD_Blockset/Signal Routing/If_Then_Else
      settings: SourceProductName=PACCAR EmE MBD Blockset
  Out1 : Outport
  wires:
  If_Then_Else/1 -> Bus Creator/1  "PedalDemToEngine"
  Inport/1 -> Bus Selector/1
  Bus Selector/2 -> Bus Creator/2, If_Then_Else/3  "<PedDrv>"
  Constant/1 -> If_Then_Else/1
  Bus Selector/1 -> If_Then_Else/2  "<APTC_arb_pedal_position>"
  Bus Creator/1 -> Out1/1

== system L4_SIM/Controllers/Virtual_Controllers/Interface_Abstraction/PICBus ==
  In : Inport
  Bus Creator : BusCreator  Inputs=4
  Bus Selector : BusSelector  OutputSignals=Feedback_sensors.Navigation.VehHeading,Operator.TargetHeading,Feedback_sensors.Chassis.VehicleSpeed,Cycle.RefVehSpeed
  Gain : Gain  Gain=pi/180.0
  Gain1 : Gain  Gain=pi/180.0
  Gain2 : Gain  Gain=1.0
  Gain3 : Gain  Gain=1.0
  Out : Outport
  wires:
  In/1 -> Bus Selector/1
  Bus Creator/1 -> Out/1
  Bus Selector/4 -> Gain3/1  "<RefVehSpeed>"
  Bus Selector/3 -> Gain2/1  "<VehicleSpeed>"
  Bus Selector/2 -> Gain1/1  "<TargetHeading>"
  Bus Selector/1 -> Gain/1  "<VehHeading>"
  Gain/1 -> Bus Creator/1  "CurrentAzimuth_rad"
  Gain1/1 -> Bus Creator/2  "TargetAzimuth_rad"
  Gain2/1 -> Bus Creator/3  "CurrentVelocity_kph"
  Gain3/1 -> Bus Creator/4  "TargetVelocity_kph"

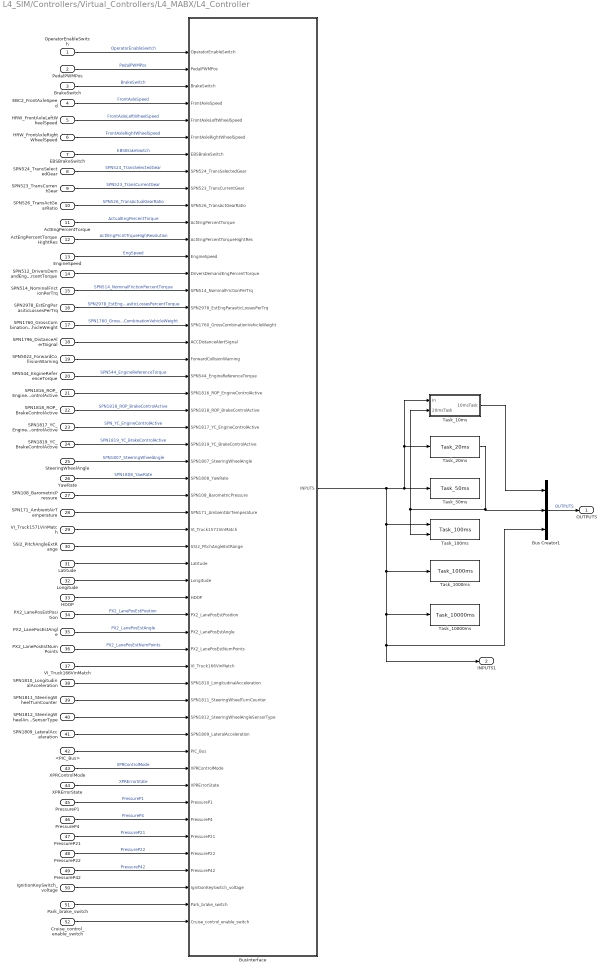
== system L4_SIM/Controllers/Virtual_Controllers/L4_MABX/L4_Controller ==
  OperatorEnableSwitch : Inport
  PedalPWMPos : Inport  Port=2
  BrakeSwitch : Inport  Port=3
  EBC2_FrontAxleSpeed : Inport  Port=4
  HRW_FrontAxleLeftWheelSpeed : Inport  Port=5
  HRW_FrontAxleRightWheelSpeed : Inport  Port=6
  EBSBrakeSwitch : Inport  Port=7
  SPN524_TransSelectedGear : Inport  Port=8
  SPN523_TransCurrentGear : Inport  Port=9
  SPN526_TransActGearRatio : Inport  Port=10
  ActEngPercentTorque : Inport  Port=11
  ActEngPercentTorqueHightRes : Inport  Port=12
  EngineSpeed : Inport  Port=13
  SPN512_DriversDemandEngPercentTorque : Inport  Port=14
  SPN514_NominalFrictionPerTrq : Inport  Port=15
  SPN2978_EstEngParasiticLossesPerTrq : Inport  Port=16
  SPN1760_GrossCombinationVehicleWeight : Inport  Port=17
  SPN1796_DistanceAlertSignal : Inport  Port=18
  SPN5022_ForwardCollisionWarning : Inport  Port=19
  SPN544_EngineReferenceTorque : Inport  Port=20
  SPN1816_ROP_EngineControlActive : Inport  Port=21
  SPN1818_ROP_BrakeControlActive : Inport  Port=22
  SPN1817_YC_EngineControlActive : Inport  Port=23
  SPN1819_YC_BrakeControlActive : Inport  Port=24
  SteeringWheelAngle : Inport  Port=25
  YawRate : Inport  Port=26
  SPN108_BarometricPressure : Inport  Port=27
  SPN171_AmbientAirTemperature : Inport  Port=28
  VI_Truck1571VinMatch : Inport  Port=29
  SSI2_PitchAngleExtRange : Inport  Port=30
  Latitude : Inport  Port=31
  Longitude : Inport  Port=32
  HDOP : Inport  Port=33
  PX2_LanePosEstPosition : Inport  Port=34
  PX2_LanePosEstAngle : Inport  Port=35
  PX2_LanePosEstNumPoints : Inport  Port=36
  VI_Truck166VinMatch : Inport  Port=37
  SPN1810_LongitudinalAcceleration : Inport  Port=38
  SPN1811_SteeringWheelTurnCounter : Inport  Port=39
  SPN1812_SteeringWheelAngleSensorType : Inport  Port=40
  SPN1809_LateralAcceleration : Inport  Port=41
  <PIC_Bus> : Inport  Port=42
  XPRControlMode : Inport  Port=43
  XPRErrorState : Inport  Port=44
  PressureP1 : Inport  Port=45
  PressureP4 : Inport  Port=46
  PressureP21 : Inport  Port=47
  PressureP22 : Inport  Port=48
  PressureP42 : Inport  Port=49
  IgnitionKeySwitch_voltage : Inport  Port=50
  Park_brake_switch : Inport  Port=51
  Cruise_control_enable_switch : Inport  Port=52
  Bus Creator1 : BusCreator  Inputs=3
  BusInterface : Subsystem
  Task_10000ms : SUB_L4_Task_10000ms/Task_10000ms
  Task_1000ms : SUB_L4_Task_1000ms/Task_1000ms
  Task_100ms : SUB_L4_Task_100ms/Task_100ms
  Task_10ms : Subsystem  AncestorBlock=SUB_L4_Task_10ms/Task_10ms  TreatAsAtomicUnit=on  SystemSampleTime=0.01
  Task_20ms : SUB_L4_Task_20ms/Task_20ms
  Task_50ms : SUB_L4_Task_50ms/Task_50ms
  OUTPUTS : Outport
  INPUTS1 : Outport  Port=2
  wires:
  PressureP42/1 -> BusInterface/49(PressureP42)  "PressureP42"
  PressureP22/1 -> BusInterface/48(PressureP22)  "PressureP22"
  PressureP21/1 -> BusInterface/47(PressureP21)  "PressureP21"
  PressureP4/1 -> BusInterface/46(PressureP4)  "PressureP4"
  PressureP1/1 -> BusInterface/45(PressureP1)  "PressureP1"
  XPRErrorState/1 -> BusInterface/44(XPRErrorState)  "XPRErrorState"
  XPRControlMode/1 -> BusInterface/43(XPRControlMode)  "XPRControlMode"
  SPN1809_LateralAcceleration/1 -> BusInterface/41(SPN1809_LateralAcceleration)
  SPN1812_SteeringWheelAngleSensorType/1 -> BusInterface/40(SPN1812_SteeringWheelAngleSensorType)
  SPN1811_SteeringWheelTurnCounter/1 -> BusInterface/39(SPN1811_SteeringWheelTurnCounter)
  SPN1810_LongitudinalAcceleration/1 -> BusInterface/38(SPN1810_LongitudinalAcceleration)
  VI_Truck166VinMatch/1 -> BusInterface/37(VI_Truck166VinMatch)
  SPN1819_YC_BrakeControlActive/1 -> BusInterface/24(SPN1819_YC_BrakeControlActive)  "SPN1819_YC_BrakeControlActive"
  SPN1817_YC_EngineControlActive/1 -> BusInterface/23(SPN1817_YC_EngineControlActive)  "SPN_YC_EngineControlActive"
  SPN1818_ROP_BrakeControlActive/1 -> BusInterface/22(SPN1818_ROP_BrakeControlActive)  "SPN1818_ROP_BrakeControlActive"
  SPN1816_ROP_EngineControlActive/1 -> BusInterface/21(SPN1816_ROP_EngineControlActive)
  YawRate/1 -> BusInterface/26(SPN1808_YawRate)  "SPN1808_YawRate"
  Task_20ms/1 -> Bus Creator1/2, Task_100ms/2, Task_10ms/2(20msTask)
  PX2_LanePosEstNumPoints/1 -> BusInterface/36(PX2_LanePosEstNumPoints)  "PX2_LanePosEstNumPoints"
  PX2_LanePosEstAngle/1 -> BusInterface/35(PX2_LanePosEstAngle)  "PX2_LanePosEstAngle"
  PX2_LanePosEstPosition/1 -> BusInterface/34(PX2_LanePosEstPosition)  "PX2_LanePosEstPosition"
  SteeringWheelAngle/1 -> BusInterface/25(SPN1807_SteeringWheelAngle)  "SPN1807_SteeringWheelAngle"
  SPN544_EngineReferenceTorque/1 -> BusInterface/20(SPN544_EngineReferenceTorque)  "SPN544_EngineReferenceTorque"
  SPN1760_GrossCombinationVehicleWeight/1 -> BusInterface/17(SPN1760_GrossCombinationVehicleWeight)  "SPN1760_GrossCombinationVehicleWeight"
  SPN2978_EstEngParasiticLossesPerTrq/1 -> BusInterface/16(SPN2978_EstEngParasiticLossesPerTrq)  "SPN2978_EstEngParasiticLossesPercentTorque"
  SPN514_NominalFrictionPerTrq/1 -> BusInterface/15(SPN514_NominalFrictionPerTrq)  "SPN514_NominalFrictionPercentTorque"
  EngineSpeed/1 -> BusInterface/13(EngineSpeed)  "EngSpeed"
  ActEngPercentTorqueHightRes/1 -> BusInterface/12(ActEngPercentTorqueHightRes)  "ActlEngPrcntTrqueHighResolution"
  ActEngPercentTorque/1 -> BusInterface/11(ActEngPercentTorque)  "ActualEngPercentTorque"
  SPN526_TransActGearRatio/1 -> BusInterface/10(SPN526_TransActGearRatio)  "SPN526_TransActualGearRatio"
  SPN523_TransCurrentGear/1 -> BusInterface/9(SPN523_TransCurrentGear)  "SPN523_TransCurrentGear"
  SPN524_TransSelectedGear/1 -> BusInterface/8(SPN524_TransSelectedGear)  "SPN524_TransSelectedGear"
  EBSBrakeSwitch/1 -> BusInterface/7(EBSBrakeSwitch)  "EBSBrakeSwitch"
  EBC2_FrontAxleSpeed/1 -> BusInterface/4(FrontAxleSpeed)  "FrontAxleSpeed"
  BrakeSwitch/1 -> BusInterface/3(BrakeSwitch)  "BrakeSwitch"
  OperatorEnableSwitch/1 -> BusInterface/1(OperatorEnableSwitch)  "OperatorEnableSwitch"
  BusInterface/1(INPUTS) -> Task_50ms/1, Task_20ms/1, Task_10ms/1(In), Task_100ms/1, Task_1000ms/1, Task_10000ms/1, Bus Creator1/3, INPUTS1/1
  Task_10ms/1(10msTask) -> Bus Creator1/1
  Bus Creator1/1 -> OUTPUTS/1  "OUTPUTS"
  SPN108_BarometricPressure/1 -> BusInterface/27(SPN108_BarometricPressure)
  SPN171_AmbientAirTemperature/1 -> BusInterface/28(SPN171_AmbientAirTemperature)
  VI_Truck1571VinMatch/1 -> BusInterface/29(VI_Truck1571VinMatch)
  SSI2_PitchAngleExtRange/1 -> BusInterface/30(SSI2_PitchAngleExtRange)
  PedalPWMPos/1 -> BusInterface/2(PedalPWMPos)  "PedalPWMPos"
  HRW_FrontAxleLeftWheelSpeed/1 -> BusInterface/5(FrontAxleLeftWheelSpeed)  "FrontAxleLeftWheelSpeed"
  HRW_FrontAxleRightWheelSpeed/1 -> BusInterface/6(FrontAxleRightWheelSpeed)  "FrontAxleRightWheelSpeed"
  Latitude/1 -> BusInterface/31(Latitude)
  Longitude/1 -> BusInterface/32(Longitude)
  HDOP/1 -> BusInterface/33(HDOP)
  SPN1796_DistanceAlertSignal/1 -> BusInterface/18(ACCDistanceAlertSignal)
  SPN5022_ForwardCollisionWarning/1 -> BusInterface/19(ForwardCollisionWarning)
  SPN512_DriversDemandEngPercentTorque/1 -> BusInterface/14(DriversDemandEngPercentTorque)
  <PIC_Bus>/1 -> BusInterface/42(PIC_Bus)
  IgnitionKeySwitch_voltage/1 -> BusInterface/50(IgnitionKeySwitch_voltage)
  Park_brake_switch/1 -> BusInterface/51(Park_brake_switch)
  Cruise_control_enable_switch/1 -> BusInterface/52(Cruise_control_enable_switch)

== system L4_SIM/Controllers/Virtual_Controllers/PCI/TSC Engine Arbitration ==
  CrsTrqDem : Inport  Unit=%/100
  PedDvr : Inport  Port=2  Unit=%/100
  TSC1_P32_BE : Inport  Port=3
  TSC1_P32_TE : Inport  Port=4
  TSC1_P4_VECU : Inport  Port=5
  TSC1_P2_VEMCE : Inport  Port=6
  TSC1_P5_ERAD : Inport  Port=7
  Bus Selector : BusSelector  OutputSignals=TrqReqE,OCME
  Bus Selector1 : BusSelector  OutputSignals=TrqReqE,OCME
  Bus Selector2 : BusSelector  OutputSignals=TrqReq,OCM
  Bus Selector3 : BusSelector  OutputSignals=TrqReqE,OCME
  Bus Selector4 : BusSelector  OutputSignals=TrqReq,OCM
  Compare To Constant : simulink/Logic and Bit Operations/Compare To Constant  relop===  const=3  OutDataTypeStr=boolean
  Compare To Constant1 : simulink/Logic and Bit Operations/Compare To Constant  relop===  const=2  OutDataTypeStr=boolean
  Compare To Constant2 : simulink/Logic and Bit Operations/Compare To Constant  relop===  const=3  OutDataTypeStr=boolean
  Compare To Constant3 : simulink/Logic and Bit Operations/Compare To Constant  relop===  const=3  OutDataTypeStr=boolean
  Compare To Constant4 : simulink/Logic and Bit Operations/Compare To Constant  relop===  const=2  OutDataTypeStr=boolean
  Compare To Constant5 : simulink/Logic and Bit Operations/Compare To Constant  relop===  const=2  OutDataTypeStr=boolean
  Constant : Constant  Value=0
  Constant2 : Constant  Value=1.25
  Gain1 : Gain  Gain=100
  MinMax : MinMax  Inputs=2
  MinMax1 : MinMax  Function=max  Inputs=3
  Switch{,1..5} (6 alike) : Switch  Criteria=u2 ~= 0
  TrqLimitABS : MinMax  Inputs=2
  TrqLimitTCM : MinMax  Inputs=2
  DriverDemPercentTrq : Outport
  EngTrqDemand : Outport  Port=2
  wires:
  CrsTrqDem/1 -> MinMax1/2
  MinMax1/1 -> MinMax/1
  PedDvr/1 -> MinMax1/1
  TSC1_P4_VECU/1 -> Bus Selector4/1
  TSC1_P2_VEMCE/1 -> Bus Selector3/1
  TSC1_P32_BE/1 -> Bus Selector/1
  TSC1_P32_TE/1 -> Bus Selector1/1
  Bus Selector1/2 -> Compare To Constant1/1, Compare To Constant/1  "<OCME>"
  Bus Selector1/1 -> Switch1/1, TrqLimitTCM/2  "<TrqReqE>"
  Compare To Constant/1 -> Switch/2
  TrqLimitTCM/1 -> Switch/1
  MinMax/1 -> Gain1/1, Switch/3, TrqLimitTCM/1
  Compare To Constant1/1 -> Switch1/2
  Bus Selector/1 -> TrqLimitABS/2  "<TrqReqE>"
  Bus Selector/2 -> Compare To Constant2/1  "<OCME>"
  Switch/1 -> Switch1/3
  Compare To Constant2/1 -> Switch2/2
  Switch1/1 -> Switch2/3, TrqLimitABS/1
  TrqLimitABS/1 -> Switch2/1
  TSC1_P5_ERAD/1 -> Bus Selector2/1
  Bus Selector2/2 -> Compare To Constant3/1  "<OCM>"
  Compare To Constant3/1 -> Switch3/2
  Bus Selector2/1 -> Switch3/1  "<TrqReq>"
  Switch2/1 -> Switch3/3
  Switch3/1 -> EngTrqDemand/1  "EngTrqDemand"
  Bus Selector3/1 -> Switch4/1  "<TrqReqE>"
  Bus Selector3/2 -> Compare To Constant4/1  "<OCME>"
  Compare To Constant4/1 -> Switch4/2
  Switch4/1 -> MinMax1/3
  Constant/1 -> Switch4/3
  Switch5/1 -> MinMax/2
  Compare To Constant5/1 -> Switch5/2
  Bus Selector4/2 -> Compare To Constant5/1  "<OCM>"
  Bus Selector4/1 -> Switch5/1  "<TrqReq>"
  Constant2/1 -> Switch5/3
  Gain1/1 -> DriverDemPercentTrq/1  "DriverDemPercentTrq"

== system L4_SIM/Controllers/Virtual_Controllers/PCI/TSC Retarder Arbitration ==
  CrsRetDem : Inport  Unit=%/100
  TSC1_P32_BR : Inport  Port=2
  TSC1_P32_TR : Inport  Port=3
  TSC1_P32_VEMCR : Inport  Port=4
  Bus Selector5 : BusSelector  OutputSignals=TrqReqR,OCMR
  Bus Selector6 : BusSelector  OutputSignals=TrqReqR,OCMR
  Bus Selector7 : BusSelector  OutputSignals=TrqReqR,OCMR
  Compare To Constant6 : simulink/Logic and Bit Operations/Compare To Constant  relop===  const=3  OutDataTypeStr=boolean
  Compare To Constant7 : simulink/Logic and Bit Operations/Compare To Constant  relop===  const=2  OutDataTypeStr=boolean
  Compare To Constant8 : simulink/Logic and Bit Operations/Compare To Constant  relop===  const=3  OutDataTypeStr=boolean
  Compare To Constant9 : simulink/Logic and Bit Operations/Compare To Constant  relop===  const=2  OutDataTypeStr=boolean
  Constant1 : Constant  Value=0
  Gain2 : Gain  Gain=100
  MinMax1 : MinMax  Function=max  Inputs=2
  Switch{6..9} (4 alike) : Switch  Criteria=u2 ~= 0
  TrqLimitABS1 : MinMax  Inputs=2
  TrqLimitTCM1 : MinMax  Inputs=2
  DriverDemandRetarderPercentTorque : Outport
  EngRetarderDemand : Outport  Port=2
  wires:
  TSC1_P32_VEMCR/1 -> Bus Selector7/1
  Bus Selector7/1 -> Switch6/1  "<TrqReqR>"
  Bus Selector7/2 -> Compare To Constant9/1  "<OCMR>"
  Compare To Constant9/1 -> Switch6/2
  Constant1/1 -> Switch6/3
  TSC1_P32_BR/1 -> Bus Selector5/1
  TSC1_P32_TR/1 -> Bus Selector6/1
  Bus Selector6/2 -> Compare To Constant7/1, Compare To Constant6/1  "<OCMR>"
  Bus Selector6/1 -> TrqLimitTCM1/2, Switch8/1  "<TrqReqR>"
  Compare To Constant6/1 -> Switch7/2
  TrqLimitTCM1/1 -> Switch7/1
  MinMax1/1 -> TrqLimitTCM1/1, Switch7/3, Gain2/1
  Compare To Constant7/1 -> Switch8/2
  Bus Selector5/1 -> TrqLimitABS1/2  "<TrqReqR>"
  Bus Selector5/2 -> Compare To Constant8/1  "<OCMR>"
  Switch7/1 -> Switch8/3
  Compare To Constant8/1 -> Switch9/2
  Switch8/1 -> Switch9/3, TrqLimitABS1/1
  TrqLimitABS1/1 -> Switch9/1
  Switch9/1 -> EngRetarderDemand/1  "EngRetarderDemand"
  Gain2/1 -> DriverDemandRetarderPercentTorque/1  "DriverDemandRetarderPercentTorque"
  CrsRetDem/1 -> MinMax1/1
  Switch6/1 -> MinMax1/2
